simulink model "simulation_test"  (R2025b)
settings: Solver=VariableStepAuto  StartTime=0.0  StopTime=50  RelTol=1e-3
libraries: simulink x6, SignalEditorBlockLib x3
settings Model: Creator=David  LastModifiedBy=David

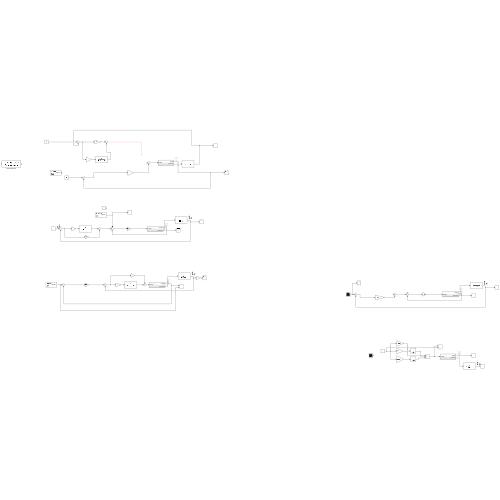
[thumbnail: Simulink's stored preview of the top-level diagram]
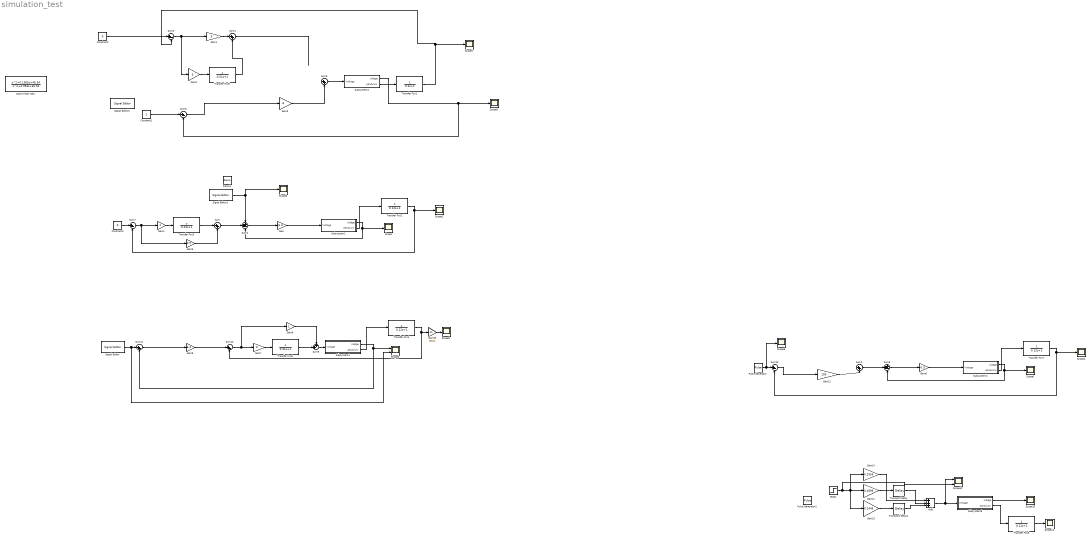
== system simulation_test ==
  Add : Sum  Inputs=+++
  Constant1 : Constant
  Constant2 : Constant  Value=0
  Constant3 : Constant  Value=0
  Gain : Gain  Gain=6.3
  Gain1 : Gain  Gain=5
  Gain10 : Gain  Gain=180/pi
  Gain11 : Gain  Gain=0.4999
  Gain12 : Gain  Gain=100
  Gain13 : Gain  Gain=0.2445
  Gain14 : Gain  Gain=0.2555
  Gain2 : Gain  Gain=5
  Gain3 : Gain  Gain=4
  Gain4 : Gain
  Gain5 : Gain  Gain=0.5
  Gain6 : Gain  Gain=6.3
  Gain7 : Gain  Gain=0
  Gain8 : Gain  Gain=6.3
  Gain9 : Gain
  Notch Filter New : TransferFcn  Numerator=[1 0.1365 46.54]  Denominator=[1 4.094 46.54]
  Pulse Generator : DiscretePulseGenerator  PulseType=Time based  Period=100  PulseWidth=0.1
  Pulse Generator2 : DiscretePulseGenerator  PulseType=Time based  Amplitude=2  Period=50  PulseWidth=5
  Ramp1 : simulink/Sources/Ramp  slope=0.1  start=0  InitialOutput=0
  Scope{,1..5,7..11} (11 alike) : Scope
      Scope settings: ActiveDisplayYMinimum=-1  ActiveDisplayYMaximum=1  DataLoggingVariableName=ScopeData3
      Scope1 settings: ActiveDisplayYMinimum=-0.95827367892618764  ActiveDisplayYMaximum=8.6244631103356912
      Scope10 settings: ActiveDisplayYMinimum=-0.058865643749571823  ActiveDisplayYMaximum=0.52979079374614657  DataLoggingVariableName=ScopeData11
      Scope11 settings: ActiveDisplayYMinimum=-0.32026877714536389  ActiveDisplayYMaximum=0.31260089525923856  DataLoggingVariableName=ScopeData14
      Scope2 settings: ActiveDisplayYMinimum=-0.099353149182499184  ActiveDisplayYMaximum=0.10092415133464305  DataLoggingVariableName=ScopeData4
      Scope3 settings: ActiveDisplayYMinimum=-0.11697351805468582  ActiveDisplayYMaximum=1.0527616624921727  DataLoggingVariableName=ScopeData6
      Scope4 settings: ActiveDisplayYMinimum=-0.32026877714536389  ActiveDisplayYMaximum=0.31260089525923856  DataLoggingVariableName=ScopeData8
      Scope5 settings: ActiveDisplayYMinimum=-0.12391597924848512  ActiveDisplayYMaximum=1.1152438132363662  DataLoggingVariableName=ScopeData5
      Scope7 settings: ActiveDisplayYMinimum=-0.050496125876241006  ActiveDisplayYMaximum=0.071160478587436973  DataLoggingVariableName=ScopeData7
      Scope8 settings: ActiveDisplayYMinimum=-0.12499999999999997  ActiveDisplayYMaximum=1.125  DataLoggingVariableName=ScopeData9
      Scope9 settings: ActiveDisplayYMinimum=-11.511569655854222  ActiveDisplayYMaximum=10.6000175606517  DataLoggingVariableName=ScopeData13
  Scope12 : Scope  NumInputPorts=2
      settings: ActiveDisplayYMinimum=-0.73844368737578758  ActiveDisplayYMaximum=6.6459931863820891  DataLoggingVariableName=ScopeData15
  Scope6 : Scope  NumInputPorts=2
      settings: ActiveDisplayYMinimum=-1  ActiveDisplayYMaximum=1  DataLoggingVariableName=ScopeData12
  Signal Editor : SignalEditorBlockLib/Signal Editor  FileName=C:\Users\David\Documents\MATLAB\cranny\signals\following.mat  ActiveScenario=Scenario  ActiveSignal=Signal 1  IsBus=off  OutputBusObjectStr=Bus: BusObject  SampleTime=0  ZeroCross=off  OutputAfterFinalValue=Setting to zero  Unit=inherit  PreserveSignalName=on  ApplySigPropsToAllScenarios=on  ApplySigPropsToAllSignals=off  SignalPropertySource=Dialog parameters
  Signal Editor1 : SignalEditorBlockLib/Signal Editor  FileName=C:\Users\David\Documents\MATLAB\cranny\signals\following.mat  ActiveScenario=Scenario  ActiveSignal=Signal 1  IsBus=off  OutputBusObjectStr=Bus: BusObject  SampleTime=0  ZeroCross=off  OutputAfterFinalValue=Setting to zero  Unit=inherit  PreserveSignalName=on  ApplySigPropsToAllScenarios=on  ApplySigPropsToAllSignals=off  SignalPropertySource=Dialog parameters
  Signal Editor2 : SignalEditorBlockLib/Signal Editor  FileName=C:\Users\David\Documents\MATLAB\cranny\signals\following.mat  ActiveScenario=Scenario  ActiveSignal=Signal 1  IsBus=off  OutputBusObjectStr=Bus: BusObject  SampleTime=0  ZeroCross=off  OutputAfterFinalValue=Setting to zero  Unit=inherit  PreserveSignalName=on  ApplySigPropsToAllScenarios=on  ApplySigPropsToAllSignals=off  SignalPropertySource=Dialog parameters
  Step1 : Step  Time=2  SampleTime=0
  Subsystem1 : Subsystem
  Subsystem2 : Subsystem
  Subsystem3 : Subsystem
  Subsystem4 : Subsystem
  Subsystem6 : Subsystem
  Sum{,1,4..5} (4 alike) : Sum  Inputs=|++
  Sum{3,6..7,10..12} (6 alike) : Sum  Inputs=|+-
  Sum2 : Sum  Inputs=++-
  Sum8 : Sum  Inputs=++-
  Sum9 : Sum  Inputs=++|
  Transfer Fcn1 : TransferFcn  Denominator=[0.2 1]
  Transfer Fcn{2,4,7..8} (4 alike) : TransferFcn  Denominator=[0.12 1]
  Transfer Fcn3 : TransferFcn  Numerator=[1 0]  Denominator=[0.01 1]
  Transfer Fcn5 : TransferFcn  Numerator=[1 0]  Denominator=[0.01 1]
  Transfer Fcn6 : TransferFcn  Numerator=[1 0]  Denominator=[0.01 1]
  Transport Delay : TransportDelay  DelayTime=0.4605
  Transport Delay1 : TransportDelay  DelayTime=0.9210
  wires:
  Gain1/1 -> Sum4/1
  Subsystem3/1(sledge) -> Scope5/1, Sum6/2
  Constant2/1 -> Sum3/1
  Subsystem3/2(pendulum) -> Transfer Fcn1/1
  Gain3/1 -> Sum5/2
  Constant1/1 -> Sum6/1
  Sum6/1 -> Gain3/1
  Sum3/1 -> Gain2/1, Gain1/1
  Gain2/1 -> Transfer Fcn5/1
  Transfer Fcn5/1 -> Sum4/2
  Sum4/1 -> ?
  Sum5/1 -> Subsystem3/1(Voltage)
  Transfer Fcn1/1 -> Sum3/2, Scope7/1
  Sum2/1 -> Gain/1
  Subsystem1/2(pendulum) -> Transfer Fcn2/1
  Subsystem1/1(sledge) -> Sum2/3, Scope/1
  Signal Editor1/1 -> Sum2/1, Scope3/1
  Gain/1 -> Subsystem1/1(Voltage)
  Gain4/1 -> Transfer Fcn3/1
  Transfer Fcn3/1 -> Sum/1
  Sum/1 -> Sum2/2
  Gain5/1 -> Sum/2
  Sum7/1 -> Gain5/1, Gain4/1
  Constant3/1 -> Sum7/1
  Transfer Fcn2/1 -> Scope2/1, Sum7/2
  Subsystem4/2(pendulum) -> Transfer Fcn4/1
  Signal Editor/1 -> Scope6/2, Sum11/1
  Sum11/1 -> Gain8/1
  Subsystem4/1(sledge) -> Sum11/2, Scope6/1
  Sum9/1 -> Subsystem4/1(Voltage)
  Transfer Fcn4/1 -> Sum10/2, Gain10/1
  Sum10/1 -> Gain9/1, Gain7/1
  Transfer Fcn6/1 -> Sum9/2
  Gain9/1 -> Sum9/1
  Gain7/1 -> Transfer Fcn6/1
  Gain8/1 -> Sum10/1
  Gain10/1 -> Scope9/1
  Subsystem2/2(pendulum) -> Transfer Fcn7/1
  Gain12/1 -> Sum1/2
  Pulse Generator/1 -> Scope8/1, Sum12/1
  Sum1/1 -> Sum8/2
  Sum12/1 -> Gain12/1
  Subsystem2/1(sledge) -> Sum8/3, Scope1/1
  Gain6/1 -> Subsystem2/1(Voltage)
  Sum8/1 -> Gain6/1
  Transfer Fcn7/1 -> Scope4/1, Sum12/2
  Gain13/1 -> Transport Delay1/1
  Gain11/1 -> Transport Delay/1
  Gain14/1 -> Add/1
  Add/1 -> Scope12/1, Subsystem6/1(Voltage)
  Transport Delay/1 -> Add/2
  Transport Delay1/1 -> Add/3
  Step1/1 -> Scope12/2, Gain13/1, Gain14/1, Gain11/1
  Subsystem6/2(pendulum) -> Transfer Fcn8/1
  Subsystem6/1(sledge) -> Scope10/1
  Transfer Fcn8/1 -> Scope11/1

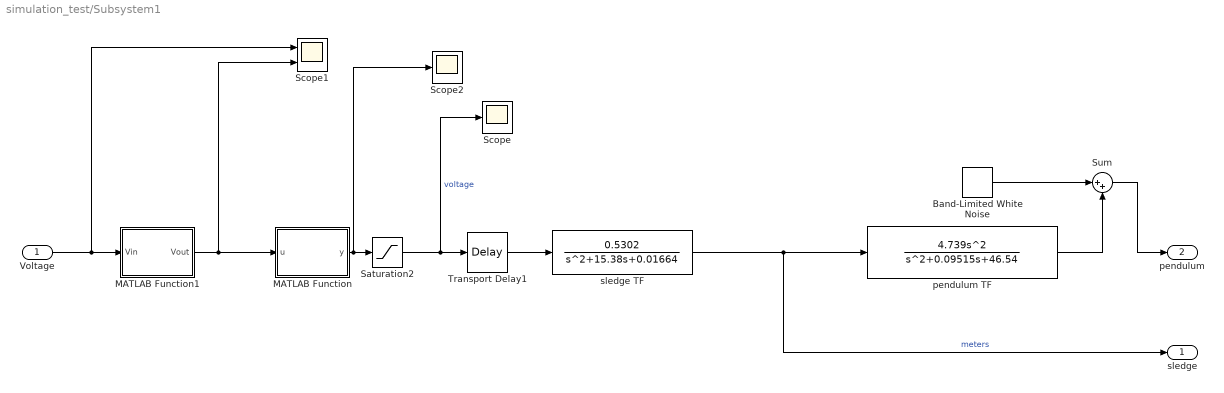
== system simulation_test/Subsystem1 ==
  Voltage : Inport
  Band-Limited White Noise : simulink/Sources/Band-Limited White Noise  Cov=[4.9008e-09]  Ts=0.01  seed=[23341]
  MATLAB Function : MATLAB Function  TreatAsAtomicUnit=on
  MATLAB Function1 : MATLAB Function  TreatAsAtomicUnit=on
  Saturation2 : Saturate  UpperLimit=16  LowerLimit=-16
  Scope : Scope
      settings: ActiveDisplayYMinimum=-1  ActiveDisplayYMaximum=1
  Scope1 : Scope  NumInputPorts=2
      settings: ActiveDisplayYMinimum=-5  ActiveDisplayYMaximum=5  DataLoggingVariableName=ScopeData2
  Scope2 : Scope
      settings: ActiveDisplayYMinimum=-1  ActiveDisplayYMaximum=1  DataLoggingVariableName=ScopeData10
  Sum : Sum  Inputs=|++
  Transport Delay1 : TransportDelay  DelayTime=0.02
  pendulum TF : TransferFcn  Numerator=[4.739 0 0]  Denominator=[1 0.09515 46.54]
  sledge TF : TransferFcn  Numerator=[0.5302]  Denominator=[1 15.38 0.01664]
  sledge : Outport
  pendulum : Outport  Port=2
  wires:
  MATLAB Function/1(y) -> Scope2/1, Saturation2/1
  MATLAB Function1/1(Vout) -> MATLAB Function/1(u), Scope1/2
  Sum/1 -> pendulum/1
  Band-Limited White Noise/1 -> Sum/1
  Transport Delay1/1 -> sledge TF/1
  pendulum TF/1 -> Sum/2
  Voltage/1 -> MATLAB Function1/1(Vin), Scope1/1
  sledge TF/1 -> sledge/1, pendulum TF/1  "meters"
  Saturation2/1 -> Transport Delay1/1, Scope/1  "voltage"

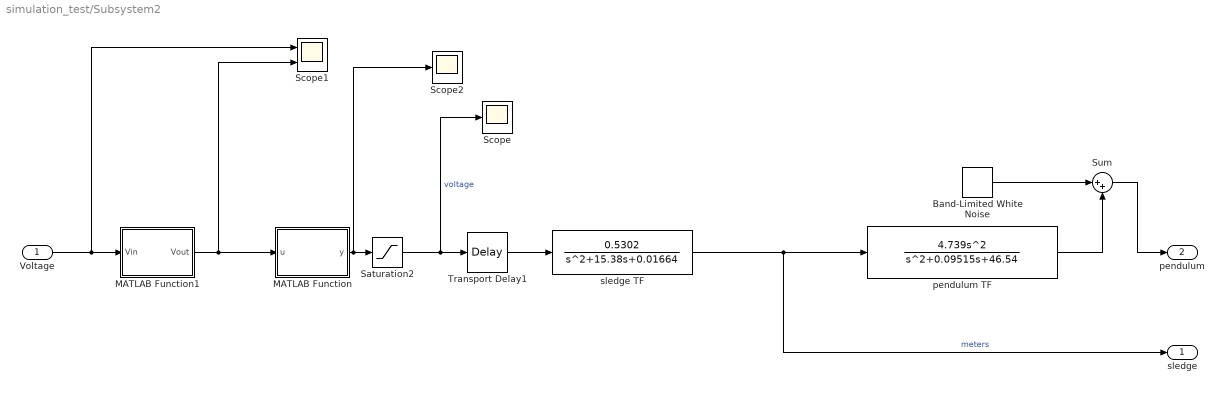
== system simulation_test/Subsystem2 ==
  Voltage : Inport
  Band-Limited White Noise : simulink/Sources/Band-Limited White Noise  Cov=[4.9008e-09]  Ts=0.01  seed=[23341]
  MATLAB Function : MATLAB Function  TreatAsAtomicUnit=on
  MATLAB Function1 : MATLAB Function  TreatAsAtomicUnit=on
  Saturation2 : Saturate  UpperLimit=16  LowerLimit=-16
  Scope : Scope
      settings: ActiveDisplayYMinimum=-6.5  ActiveDisplayYMaximum=18.5
  Scope1 : Scope  NumInputPorts=2
      settings: ActiveDisplayYMinimum=-5  ActiveDisplayYMaximum=5  DataLoggingVariableName=ScopeData2
  Scope2 : Scope
      settings: ActiveDisplayYMinimum=-1  ActiveDisplayYMaximum=1  DataLoggingVariableName=ScopeData10
  Sum : Sum  Inputs=|++
  Transport Delay1 : TransportDelay  DelayTime=0.02
  pendulum TF : TransferFcn  Numerator=[4.739 0 0]  Denominator=[1 0.09515 46.54]
  sledge TF : TransferFcn  Numerator=[0.5302]  Denominator=[1 15.38 0.01664]
  sledge : Outport
  pendulum : Outport  Port=2
  wires:
  MATLAB Function/1(y) -> Scope2/1, Saturation2/1
  MATLAB Function1/1(Vout) -> MATLAB Function/1(u), Scope1/2
  Sum/1 -> pendulum/1
  Band-Limited White Noise/1 -> Sum/1
  Transport Delay1/1 -> sledge TF/1
  pendulum TF/1 -> Sum/2
  Voltage/1 -> MATLAB Function1/1(Vin), Scope1/1
  sledge TF/1 -> sledge/1, pendulum TF/1  "meters"
  Saturation2/1 -> Transport Delay1/1, Scope/1  "voltage"

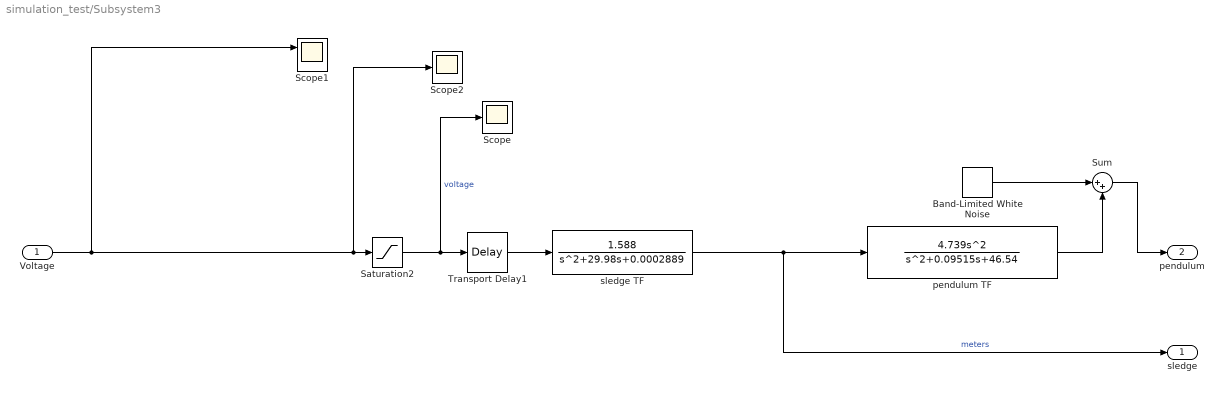
== system simulation_test/Subsystem3 ==
  Voltage : Inport
  Band-Limited White Noise : simulink/Sources/Band-Limited White Noise  Cov=[4.9008e-09]  Ts=0.01  seed=[23341]
  Saturation2 : Saturate  UpperLimit=16  LowerLimit=-16
  Scope : Scope
      settings: ActiveDisplayYMinimum=-1  ActiveDisplayYMaximum=1
  Scope1 : Scope  NumInputPorts=2
      settings: ActiveDisplayYMinimum=-5  ActiveDisplayYMaximum=5  DataLoggingVariableName=ScopeData2
  Scope2 : Scope
      settings: ActiveDisplayYMinimum=-1  ActiveDisplayYMaximum=1  DataLoggingVariableName=ScopeData10
  Sum : Sum  Inputs=|++
  Transport Delay1 : TransportDelay  DelayTime=0.02
  pendulum TF : TransferFcn  Numerator=[4.739 0 0]  Denominator=[1 0.09515 46.54]
  sledge TF : TransferFcn  Numerator=[1.588]  Denominator=[1 29.98 0.0002889]
  sledge : Outport
  pendulum : Outport  Port=2
  wires:
  Saturation2/1 -> Scope/1, Transport Delay1/1  "voltage"
  sledge TF/1 -> pendulum TF/1, sledge/1  "meters"
  pendulum TF/1 -> Sum/2
  Transport Delay1/1 -> sledge TF/1
  Band-Limited White Noise/1 -> Sum/1
  Sum/1 -> pendulum/1
  Voltage/1 -> Saturation2/1, Scope2/1, Scope1/1

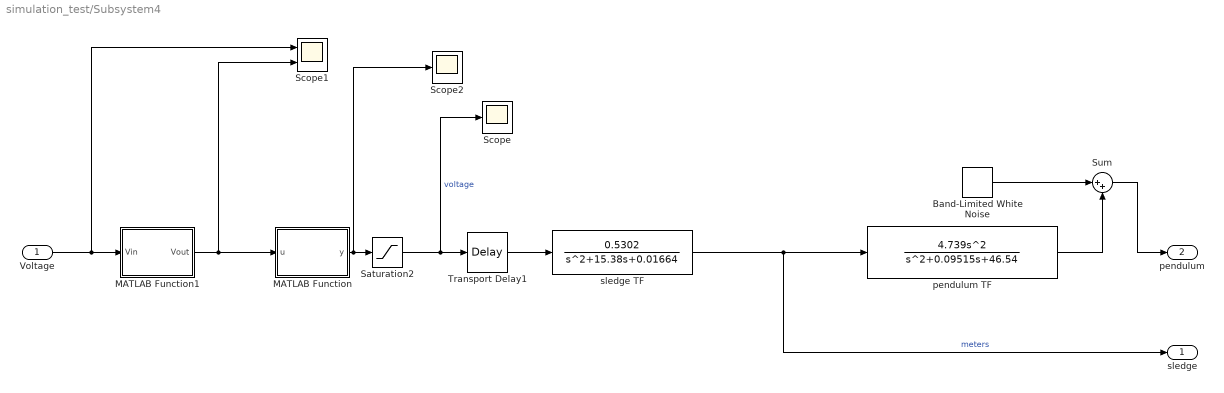
== system simulation_test/Subsystem4 ==
  Voltage : Inport
  Band-Limited White Noise : simulink/Sources/Band-Limited White Noise  Cov=[4.9008e-09]  Ts=0.01  seed=[23341]
  MATLAB Function : MATLAB Function  TreatAsAtomicUnit=on
  MATLAB Function1 : MATLAB Function  TreatAsAtomicUnit=on
  Saturation2 : Saturate  UpperLimit=16  LowerLimit=-16
  Scope : Scope
      settings: ActiveDisplayYMinimum=-1  ActiveDisplayYMaximum=1
  Scope1 : Scope  NumInputPorts=2
      settings: ActiveDisplayYMinimum=-5  ActiveDisplayYMaximum=5  DataLoggingVariableName=ScopeData2
  Scope2 : Scope
      settings: ActiveDisplayYMinimum=-1  ActiveDisplayYMaximum=1  DataLoggingVariableName=ScopeData10
  Sum : Sum  Inputs=|++
  Transport Delay1 : TransportDelay  DelayTime=0.02
  pendulum TF : TransferFcn  Numerator=[4.739 0 0]  Denominator=[1 0.09515 46.54]
  sledge TF : TransferFcn  Numerator=[0.5302]  Denominator=[1 15.38 0.01664]
  sledge : Outport
  pendulum : Outport  Port=2
  wires:
  MATLAB Function/1(y) -> Scope2/1, Saturation2/1
  MATLAB Function1/1(Vout) -> MATLAB Function/1(u), Scope1/2
  Sum/1 -> pendulum/1
  Band-Limited White Noise/1 -> Sum/1
  Transport Delay1/1 -> sledge TF/1
  pendulum TF/1 -> Sum/2
  Voltage/1 -> MATLAB Function1/1(Vin), Scope1/1
  sledge TF/1 -> sledge/1, pendulum TF/1  "meters"
  Saturation2/1 -> Transport Delay1/1, Scope/1  "voltage"

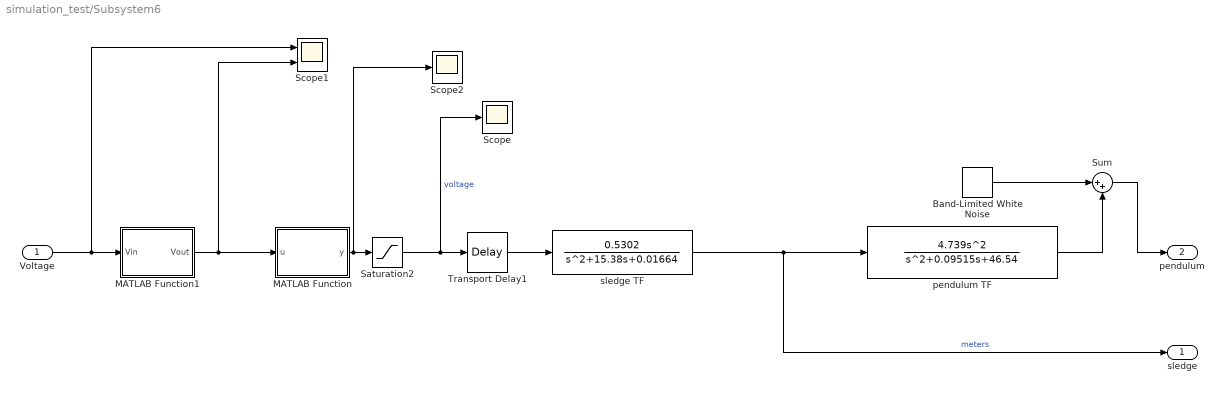
== system simulation_test/Subsystem6 ==
  Voltage : Inport
  Band-Limited White Noise : simulink/Sources/Band-Limited White Noise  Cov=[4.9008e-09]  Ts=0.01  seed=[23341]
  MATLAB Function : MATLAB Function  TreatAsAtomicUnit=on
  MATLAB Function1 : MATLAB Function  TreatAsAtomicUnit=on
  Saturation2 : Saturate  UpperLimit=16  LowerLimit=-16
  Scope : Scope
      settings: ActiveDisplayYMinimum=-6.5  ActiveDisplayYMaximum=18.5
  Scope1 : Scope  NumInputPorts=2
      settings: ActiveDisplayYMinimum=-5  ActiveDisplayYMaximum=5  DataLoggingVariableName=ScopeData2
  Scope2 : Scope
      settings: ActiveDisplayYMinimum=-1  ActiveDisplayYMaximum=1  DataLoggingVariableName=ScopeData10
  Sum : Sum  Inputs=|++
  Transport Delay1 : TransportDelay  DelayTime=0.02
  pendulum TF : TransferFcn  Numerator=[4.739 0 0]  Denominator=[1 0.09515 46.54]
  sledge TF : TransferFcn  Numerator=[0.5302]  Denominator=[1 15.38 0.01664]
  sledge : Outport
  pendulum : Outport  Port=2
  wires:
  MATLAB Function/1(y) -> Scope2/1, Saturation2/1
  MATLAB Function1/1(Vout) -> MATLAB Function/1(u), Scope1/2
  Sum/1 -> pendulum/1
  Band-Limited White Noise/1 -> Sum/1
  Transport Delay1/1 -> sledge TF/1
  pendulum TF/1 -> Sum/2
  Voltage/1 -> MATLAB Function1/1(Vin), Scope1/1
  sledge TF/1 -> sledge/1, pendulum TF/1  "meters"
  Saturation2/1 -> Transport Delay1/1, Scope/1  "voltage"

== matlab function simulation_test/Subsystem1/MATLAB Function ==
  data: u input; y output
function y = deadzone(u)
V_min = 4;

if abs(u) < V_min
    y = 0;
else
    y = u;
end

== matlab function simulation_test/Subsystem1/MATLAB Function1 ==
  data: Vin input; Vout output
function Vout = clamping(Vin)
V_min = 4;
dir = sign(Vin);

if Vin < V_min
    Vout = dir*V_min;
else
    Vout = Vin;

end

== matlab function simulation_test/Subsystem2/MATLAB Function1 ==
  data: Vin input; Vout output
function Vout = clamping(Vin)
V_min = 4;
dir = sign(Vin);

if Vin < V_min
    Vout = dir*V_min;
else
    Vout = Vin;

end

== matlab function simulation_test/Subsystem4/MATLAB Function ==
  data: u input; y output
function y = deadzone(u)
V_min = 4;

if abs(u) < V_min
    y = 0;
else
    y = u;
end

== matlab function simulation_test/Subsystem4/MATLAB Function1 ==
  data: Vin input; Vout output
function Vout = clamping(Vin)
V_min = 4;
dir = sign(Vin);

if Vin < V_min
    Vout = dir*V_min;
else
    Vout = Vin;

end

== matlab function simulation_test/Subsystem6/MATLAB Function ==
  data: u input; y output
function y = deadzone(u)
V_min = 4;

if abs(u) < V_min
    y = 0;
else
    y = u;
end

== matlab function simulation_test/Subsystem6/MATLAB Function1 ==
  data: Vin input; Vout output
function Vout = clamping(Vin)
V_min = 4;
dir = sign(Vin);

if Vin < V_min
    Vout = dir*V_min;
else
    Vout = Vin;

end

== matlab function simulation_test/Subsystem2/MATLAB Function ==
  data: u input; y output
function y = deadzone(u)
V_min = 4;

if abs(u) < V_min
    y = 0;
else
    y = u;
end
